simulink model "regulator"  (R2013b)
settings: Solver=ode3  StartTime=0.0  StopTime=9000  FixedStep=0.1  RelTol=1e-3
undefined symbols (not defined in the file): Calka, Kp, Ti, To, Tzco
libraries: simulink_extras x1
settings Model: Creator=Szymek  LastModifiedBy=Szymek
settings DataIOCC: FinalStateName=regulatorSimState  SaveFinalState=on  SaveCompleteFinalSimState=on

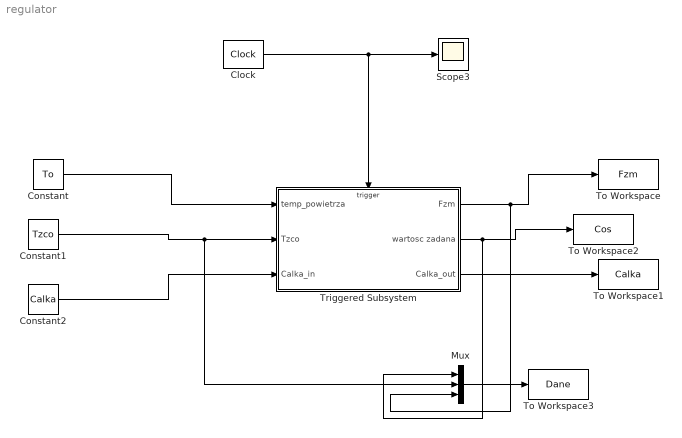
== system regulator ==
  Clock : simulink_extras/Flip Flops/Clock  period=2
  Constant : Constant  Value=To
  Constant1 : Constant  Value=Tzco
  Constant2 : Constant  Value=Calka
  Mux : Mux  Inputs=3
  Scope3 : Scope
      settings: SaveName=ScopeData3
  To Workspace : ToWorkspace  VariableName=Fzm  SampleTime=-1
      settings: MaxDataPoints=1
  To Workspace1 : ToWorkspace  VariableName=Calka  SampleTime=-1
      settings: MaxDataPoints=1
  To Workspace2 : ToWorkspace  VariableName=Cos  SampleTime=-1
      settings: MaxDataPoints=1
  To Workspace3 : ToWorkspace  VariableName=Dane  SampleTime=-1  SaveFormat=Structure With Time
  Triggered Subsystem : Subsystem  TreatAsAtomicUnit=on
  wires:
  Clock/1 -> Scope3/1, Triggered Subsystem/Trigger
  Triggered Subsystem/1(Fzm) -> Mux/3, To Workspace/1
  Triggered Subsystem/3(Calka_out) -> To Workspace1/1
  Constant/1 -> Triggered Subsystem/1(temp_powietrza)
  Constant1/1 -> Mux/2, Triggered Subsystem/2(Tzco)
  Constant2/1 -> Triggered Subsystem/3(Calka_in)
  Triggered Subsystem/2(wartosc zadana) -> Mux/1, To Workspace2/1
  Mux/1 -> To Workspace3/1

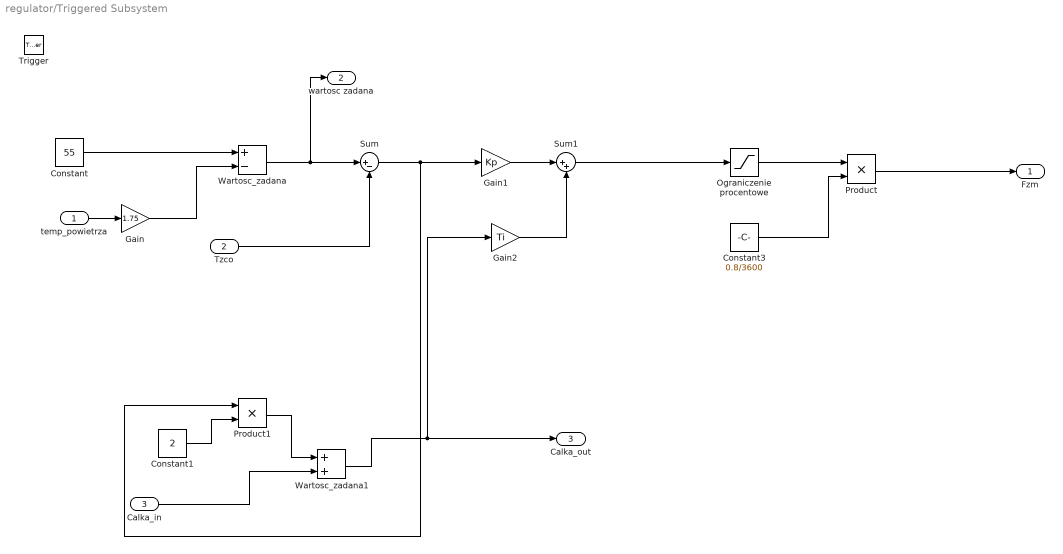
== system regulator/Triggered Subsystem ==
  temp_powietrza : Inport
  Tzco : Inport  Port=2
  Calka_in : Inport  Port=3
  Trigger : TriggerPort  PortDimensions=1
  Constant : Constant  Value=55
  Constant1 : Constant  Value=2
  Constant3 : Constant  Value=0.8/3600
  Gain : Gain  Gain=1.75
  Gain1 : Gain  Gain=Kp
  Gain2 : Gain  Gain=Ti
  Ograniczenie procentowe : Saturate  UpperLimit=100  LowerLimit=0
  Product : Product
  Product1 : Product
  Sum : Sum  Inputs=|+-
  Sum1 : Sum  Inputs=|++
  Wartosc_zadana : Sum  Inputs=+-
  Wartosc_zadana1 : Sum
  Fzm : Outport
  wartosc zadana : Outport  Port=2
  Calka_out : Outport  Port=3
  wires:
  Sum/1 -> Product1/1, Gain1/1
  Calka_in/1 -> Wartosc_zadana1/2
  Constant/1 -> Wartosc_zadana/1
  Gain/1 -> Wartosc_zadana/2
  Wartosc_zadana/1 -> wartosc zadana/1, Sum/1
  Tzco/1 -> Sum/2
  Ograniczenie procentowe/1 -> Product/1
  Constant3/1 -> Product/2
  Sum1/1 -> Ograniczenie procentowe/1
  Constant1/1 -> Product1/2
  Product1/1 -> Wartosc_zadana1/1
  Product/1 -> Fzm/1
  Gain1/1 -> Sum1/1
  temp_powietrza/1 -> Gain/1
  Gain2/1 -> Sum1/2
  Wartosc_zadana1/1 -> Gain2/1, Calka_out/1
